simulink model "soru1d"  (R2019a)
settings: Solver=VariableStepAuto  StartTime=0.0  StopTime=30  RelTol=1e-3
settings Model: Creator=handeyildirim  LastModifiedBy=handeyildirim

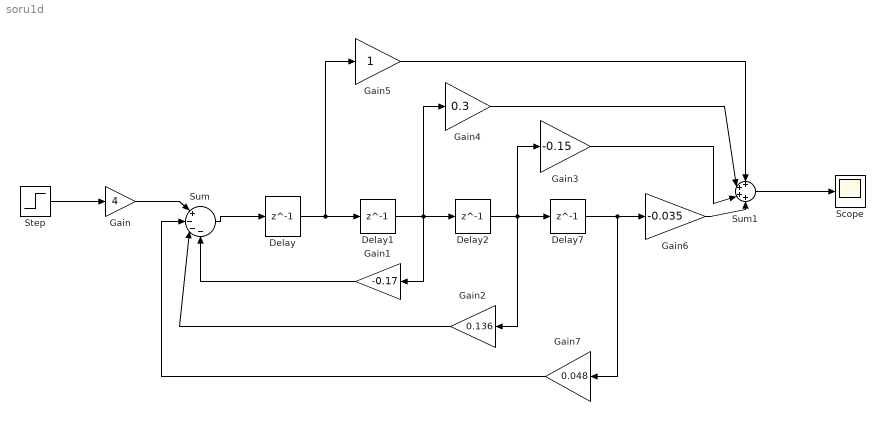
== system soru1d ==
  Delay{,1..2,7} (4 alike) : Delay  DelayLength=1
  Gain : Gain  Gain=4
  Gain1 : Gain  Gain=-0.17
  Gain2 : Gain  Gain=0.136
  Gain3 : Gain  Gain=-0.15
  Gain4 : Gain  Gain=0.3
  Gain5 : Gain
  Gain6 : Gain  Gain=-0.035
  Gain7 : Gain  Gain=0.048
  Scope : Scope
  Step : Step  SampleTime=1
  Sum : Sum  Inputs=|+---
  Sum1 : Sum  Inputs=++++
  wires:
  Step/1 -> Gain/1
  Delay/1 -> Delay1/1, Gain5/1
  Sum/1 -> Delay/1
  Delay7/1 -> Gain6/1, Gain7/1
  Delay2/1 -> Gain2/1, Delay7/1, Gain3/1
  Delay1/1 -> Gain1/1, Delay2/1, Gain4/1
  Gain1/1 -> Sum/4
  Gain/1 -> Sum/1
  Gain7/1 -> Sum/2
  Gain2/1 -> Sum/3
  Sum1/1 -> Scope/1
  Gain6/1 -> Sum1/4
  Gain3/1 -> Sum1/3
  Gain4/1 -> Sum1/2
  Gain5/1 -> Sum1/1
